simulink library "BilnrIntrpnMplXDyn"  (R2013b)
settings: Solver=ode45  StartTime=0.0  StopTime=10.0  RelTol=1e-3
settings Model: Creator=qzwc4r  LastModifiedBy=DZ1YRM

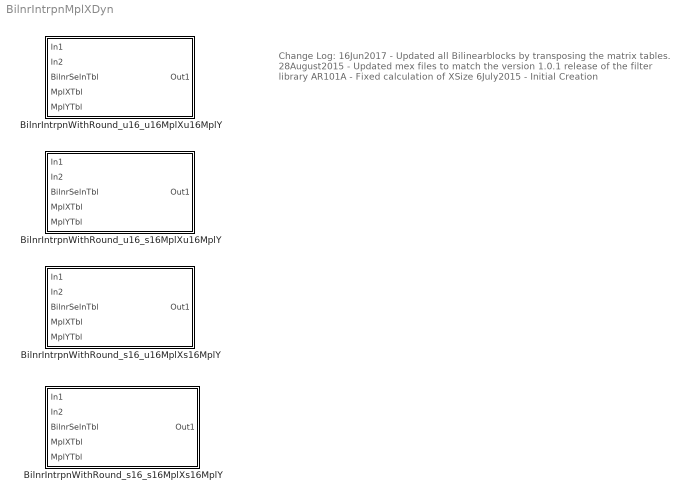
== system BilnrIntrpnMplXDyn ==
  note: Change Log:
      |
      | 16Jun2017
      | - Updated all Bilinearblocks by transposing the matrix tables.
      |
      | 28August2015
      | - Updated mex files to match the version 1.0.1 release of the filter library AR101A
      | - Fixed calculation of XSize
      |
      | 6July2015
      | - Initial Creation
  BilnrIntrpnWithRound_s16_s16MplXs16MplY : Subsystem  mask(BilnrIntrpnWithRound_s16_s16MplXs16MplY){}
      mask help: Bilinear interpolation with signed input and signed output (multiple X tables, multiple Y tables)
      settings: AttributesFormatString=Bilnr ( s16MplX , s16MplY )
      mask Display:
      | Xx = [0.45, .9];
      | Xy = [0.5, 0.5];
      | Yx = [0.6750, 0.6750];
      | Yy = [0.1, .9];
      | 
      | px = [.45, .5, .7, .75, .8, .9];
      | py1 = [.1,  .1, .3, .4, .5, .9];
      | py2 = py1+0.15;
      | py3 = py2+0.15;
      | plot(Xx,Xy, Yx,Yy, px,py1, px,py2, px,py3)
      | 
      | port_label('input',1,'Inp')
      | port_label('input',2,'BilnrSelInp')
      | port_label('input',3,'BilnrSelnTbl')
      | port_label('input',4,'MplXTbl')
      | port_label('input',5,'MplYTbl')
  BilnrIntrpnWithRound_s16_u16MplXs16MplY : Subsystem  mask(BilnrIntrpnWithRound_s16_u16MplXs16MplY){}
      mask help: Bilinear interpolation with unsigned input and signed output (multiple X tables, multiple Y tables)
      settings: AttributesFormatString=Bilnr ( u16MplX , s16MplY )
      mask Display:
      | Xx = [0.45, .9];
      | Xy = [0.4, 0.4];
      | Yx = [0.45, 0.45];
      | Yy = [0, .7];
      | 
      | px = [0.45, .5, .6, .7, .8, .9];
      | py1 = [.72, .7, .6, .3, .25, .25];
      | py2 = py1-0.1;
      | py3 = py2-0.1;
      | 
      | plot(Xx,Xy, Yx,Yy, px,py1, px,py2, px,py3)
      | 
      | port_label('input',1,'Inp')
      | port_label('input',2,'BilnrSelInp')
      | port_label('input',3,'BilnrSelnTbl')
      | port_label('input',4,'MplXTbl')
      | port_label('input',5,'MplYTbl')
  BilnrIntrpnWithRound_u16_s16MplXu16MplY : Subsystem  mask(BilnrIntrpnWithRound_u16_s16MplXu16MplY){}
      mask help: Bilinear interpolation with signed input and unsigned output (multiple X tables, multiple Y tables)
      settings: AttributesFormatString=Bilnr ( u16MplX , u16MplY )
      mask Display:
      | Xx = [.45, .9];
      | Xy = [.05, .05];
      | Yx = [.675, .675];
      | Yy = [.05, .9];
      | 
      | px = [0.45, .5, .6, .7, .8, .9];
      | py1 = [.1, .1, .2, .5, .6, .65];
      | py2 = py1+.15;
      | py3 = py2+.15;
      | 
      | plot(Xx,Xy, Yx,Yy, px,py1, px,py2, px,py3)
      | 
      | port_label('input',1,'Inp')
      | port_label('input',2,'BilnrSelInp')
      | port_label('input',3,'BilnrSelnTbl')
      | port_label('input',4,'MplXTbl')
      | port_label('input',5,'MplYTbl')
  BilnrIntrpnWithRound_u16_u16MplXu16MplY : Subsystem  mask(BilnrIntrpnWithRound_u16_u16MplXu16MplY){}
      mask help: Bilinear interpolation with signed input and unsigned output (multiple X tables, multiple Y tables)
      settings: AttributesFormatString=Bilnr ( u16MplX , u16MplY )
      mask Display:
      | Xx = [0.45, .9];
      | Xy = [0.1, 0.1];
      | Yx = [0.45, 0.45];
      | Yy = [0.1, .7];
      | 
      | px = [0.45, .5, .55, .6, .65, .7, .9];
      | 
      | py1 = [0.1,  0.4, .6, .7, .75, .8, .8];
      | py2 = [0.1,  0.4, .5, .6, .65, .7, .7];
      | py3 = [0.1,  0.3, .4, .5, .55, .6, .6];
      | 
      | plot(Xx,Xy, Yx,Yy, px,py1, px,py2, px,py3)
      | 
      | port_label('input',1,'Inp')
      | port_label('input',2,'BilnrSelInp')
      | port_label('input',3,'BilnrSelnTbl')
      | port_label('input',4,'MplXTbl')
      | port_label('input',5,'MplYTbl')

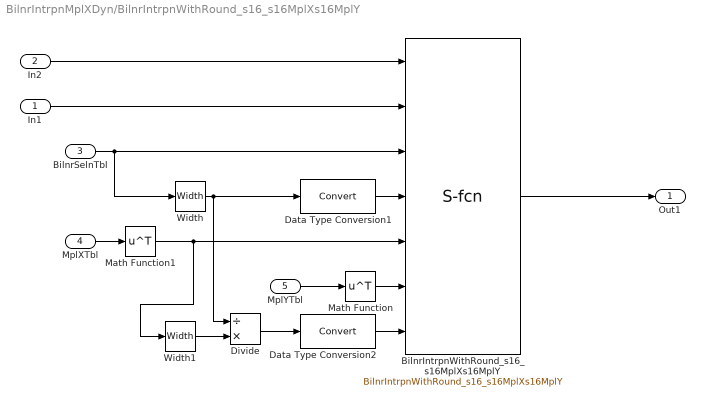
== system BilnrIntrpnMplXDyn/BilnrIntrpnWithRound_s16_s16MplXs16MplY ==
  In1 : Inport
  In2 : Inport  Port=2
  BilnrSelnTbl : Inport  Port=3
  MplXTbl : Inport  Port=4
  MplYTbl : Inport  Port=5
  BilnrIntrpnWithRound_s16_s16MplXs16MplY : S-Function  FunctionName=BilnrIntrpnWithRound_s16_s16MplXs16MplY  EnableBusSupport=off  mask(Legacy Function){SFunctionSpec=int16 y1 = BilnrIntrpnWithRound_s16_s16MplXs16MplY(uint16 u1,  int16 u2, uint16 u3[], uint16 u4,  int16 u5[],  int16 u6[], uint16 u7), ShowSpec=off}
      mask prompts: ShowSpec "Display function specification"
      mask help:
      | This block allows you to call the legacy functions specified by the following Legacy Code Tool definition:
      | def.SFunctionName = 'BilnrIntrpnWithRound_s16_s16MplXs16MplY';
      | def.OutputFcnSpec = ' int16 y1 = BilnrIntrpnWithRound_s16_s16MplXs16MplY(uint16 u1,  int16 u2, uint16 u3[], uint16 u4,  int16 u5[],  int16 u6[], uint16 u7)';
      | def.HeaderFiles = {'NxtrIntrpn.h', 'NxtrIntrpn_MemMap.h', 'Std_Types.h', 'Platform_Types.h', 'Compiler.h', 'Compiler_Cfg.h'};
      | def.SourceFiles = {'NxtrIntrpn.c'};
      | def.IncPaths = {'..\SrcFiles'};
      | def.SrcPaths = {'..\SrcFiles'};
      mask Help: <p>This block was generated automatically by the Legacy Code Tool. For detailed help on this tool, call<a href="matlab:legacy_code('help')"> legacy_code('help')</a>.</p>
      mask Callback ShowSpec:
      | if strcmp(get_param(gcbh, 'ShowSpec'), 'on')
      |   set_param(gcbh, 'MaskDisplay', sprintf('fprintf(''%s'');', get_param(gcbh, 'SFunctionSpec')));
      | else
      |   set_param(gcbh, 'MaskDisplay', sprintf('fprintf(''%s'');', get_param(gcbh, 'FunctionName')));
      | end
      mask Display: fprintf('%s',' int16 y1 = BilnrIntrpnWithRound_s16_s16MplXs16MplY(uint16 u1,  int16 u2, uint16 u3[], uint16 u4,  int16 u5[],  int16 u6[], uint16 u7)');
  Data Type Conversion1 : DataTypeConversion
  Data Type Conversion2 : DataTypeConversion
  Divide : Product  Inputs=/*
  Math Function : Math  Operator=transpose  SaturateOnIntegerOverflow=on
  Math Function1 : Math  Operator=transpose  SaturateOnIntegerOverflow=on
  Width : Width
  Width1 : Width
  Out1 : Outport
  wires:
  Width/1 -> Data Type Conversion1/1, Divide/1
  BilnrSelnTbl/1 -> Width/1, BilnrIntrpnWithRound_s16_s16MplXs16MplY/3
  In2/1 -> BilnrIntrpnWithRound_s16_s16MplXs16MplY/1
  MplYTbl/1 -> Math Function/1
  BilnrIntrpnWithRound_s16_s16MplXs16MplY/1 -> Out1/1
  In1/1 -> BilnrIntrpnWithRound_s16_s16MplXs16MplY/2
  Data Type Conversion1/1 -> BilnrIntrpnWithRound_s16_s16MplXs16MplY/4
  Data Type Conversion2/1 -> BilnrIntrpnWithRound_s16_s16MplXs16MplY/7
  MplXTbl/1 -> Math Function1/1
  Width1/1 -> Divide/2
  Divide/1 -> Data Type Conversion2/1
  Math Function/1 -> BilnrIntrpnWithRound_s16_s16MplXs16MplY/6
  Math Function1/1 -> BilnrIntrpnWithRound_s16_s16MplXs16MplY/5, Width1/1

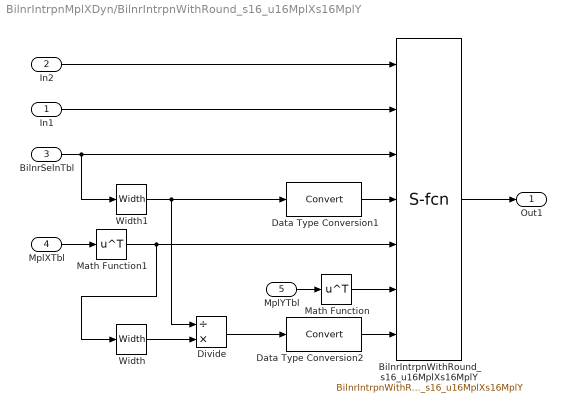
== system BilnrIntrpnMplXDyn/BilnrIntrpnWithRound_s16_u16MplXs16MplY ==
  In1 : Inport
  In2 : Inport  Port=2
  BilnrSelnTbl : Inport  Port=3
  MplXTbl : Inport  Port=4
  MplYTbl : Inport  Port=5
  BilnrIntrpnWithRound_s16_u16MplXs16MplY : S-Function  FunctionName=BilnrIntrpnWithRound_s16_u16MplXs16MplY  EnableBusSupport=off  mask(Legacy Function){SFunctionSpec=int16 y1 = BilnrIntrpnWithRound_s16_u16MplXs16MplY(uint16 u1, uint16 u2, uint16 u3[], uint16 u4, uint16 u5[],  int16 u6[], uint16 u7), ShowSpec=off}
      mask prompts: ShowSpec "Display function specification"
      mask help:
      | This block allows you to call the legacy functions specified by the following Legacy Code Tool definition:
      | def.SFunctionName = 'BilnrIntrpnWithRound_s16_u16MplXs16MplY';
      | def.OutputFcnSpec = ' int16 y1 = BilnrIntrpnWithRound_s16_u16MplXs16MplY(uint16 u1, uint16 u2, uint16 u3[], uint16 u4, uint16 u5[],  int16 u6[], uint16 u7)';
      | def.HeaderFiles = {'NxtrIntrpn.h', 'NxtrIntrpn_MemMap.h', 'Std_Types.h', 'Platform_Types.h', 'Compiler.h', 'Compiler_Cfg.h'};
      | def.SourceFiles = {'NxtrIntrpn.c'};
      | def.IncPaths = {'..\SrcFiles'};
      | def.SrcPaths = {'..\SrcFiles'};
      mask Help: <p>This block was generated automatically by the Legacy Code Tool. For detailed help on this tool, call<a href="matlab:legacy_code('help')"> legacy_code('help')</a>.</p>
      mask Callback ShowSpec:
      | if strcmp(get_param(gcbh, 'ShowSpec'), 'on')
      |   set_param(gcbh, 'MaskDisplay', sprintf('fprintf(''%s'');', get_param(gcbh, 'SFunctionSpec')));
      | else
      |   set_param(gcbh, 'MaskDisplay', sprintf('fprintf(''%s'');', get_param(gcbh, 'FunctionName')));
      | end
      mask Display: fprintf('%s',' int16 y1 = BilnrIntrpnWithRound_s16_u16MplXs16MplY(uint16 u1, uint16 u2, uint16 u3[], uint16 u4, uint16 u5[],  int16 u6[], uint16 u7)');
  Data Type Conversion1 : DataTypeConversion
  Data Type Conversion2 : DataTypeConversion
  Divide : Product  Inputs=/*
  Math Function : Math  Operator=transpose  SaturateOnIntegerOverflow=on
  Math Function1 : Math  Operator=transpose  SaturateOnIntegerOverflow=on
  Width : Width
  Width1 : Width
  Out1 : Outport
  wires:
  BilnrSelnTbl/1 -> BilnrIntrpnWithRound_s16_u16MplXs16MplY/3, Width1/1
  In2/1 -> BilnrIntrpnWithRound_s16_u16MplXs16MplY/1
  BilnrIntrpnWithRound_s16_u16MplXs16MplY/1 -> Out1/1
  In1/1 -> BilnrIntrpnWithRound_s16_u16MplXs16MplY/2
  Width1/1 -> Divide/1, Data Type Conversion1/1
  Data Type Conversion1/1 -> BilnrIntrpnWithRound_s16_u16MplXs16MplY/4
  Data Type Conversion2/1 -> BilnrIntrpnWithRound_s16_u16MplXs16MplY/7
  MplXTbl/1 -> Math Function1/1
  MplYTbl/1 -> Math Function/1
  Divide/1 -> Data Type Conversion2/1
  Width/1 -> Divide/2
  Math Function/1 -> BilnrIntrpnWithRound_s16_u16MplXs16MplY/6
  Math Function1/1 -> BilnrIntrpnWithRound_s16_u16MplXs16MplY/5, Width/1

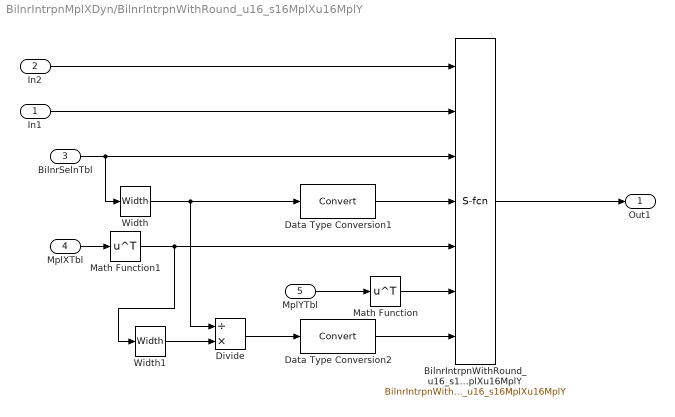
== system BilnrIntrpnMplXDyn/BilnrIntrpnWithRound_u16_s16MplXu16MplY ==
  In1 : Inport
  In2 : Inport  Port=2
  BilnrSelnTbl : Inport  Port=3
  MplXTbl : Inport  Port=4
  MplYTbl : Inport  Port=5
  BilnrIntrpnWithRound_u16_s16MplXu16MplY : S-Function  FunctionName=BilnrIntrpnWithRound_u16_s16MplXu16MplY  EnableBusSupport=off  mask(Legacy Function){SFunctionSpec=uint16 y1 = BilnrIntrpnWithRound_u16_s16MplXu16MplY(uint16 u1,  int16 u2, uint16 u3[], uint16 u4,  int16 u5[], uint16 u6[], uint16 u7), ShowSpec=off}
      mask prompts: ShowSpec "Display function specification"
      mask help:
      | This block allows you to call the legacy functions specified by the following Legacy Code Tool definition:
      | def.SFunctionName = 'BilnrIntrpnWithRound_u16_s16MplXu16MplY';
      | def.OutputFcnSpec = 'uint16 y1 = BilnrIntrpnWithRound_u16_s16MplXu16MplY(uint16 u1,  int16 u2, uint16 u3[], uint16 u4,  int16 u5[], uint16 u6[], uint16 u7)';
      | def.HeaderFiles = {'NxtrIntrpn.h', 'NxtrIntrpn_MemMap.h', 'Std_Types.h', 'Platform_Types.h', 'Compiler.h', 'Compiler_Cfg.h'};
      | def.SourceFiles = {'NxtrIntrpn.c'};
      | def.IncPaths = {'..\SrcFiles'};
      | def.SrcPaths = {'..\SrcFiles'};
      mask Help: <p>This block was generated automatically by the Legacy Code Tool. For detailed help on this tool, call<a href="matlab:legacy_code('help')"> legacy_code('help')</a>.</p>
      mask Callback ShowSpec:
      | if strcmp(get_param(gcbh, 'ShowSpec'), 'on')
      |   set_param(gcbh, 'MaskDisplay', sprintf('fprintf(''%s'');', get_param(gcbh, 'SFunctionSpec')));
      | else
      |   set_param(gcbh, 'MaskDisplay', sprintf('fprintf(''%s'');', get_param(gcbh, 'FunctionName')));
      | end
      mask Display: fprintf('%s','uint16 y1 = BilnrIntrpnWithRound_u16_s16MplXu16MplY(uint16 u1,  int16 u2, uint16 u3[], uint16 u4,  int16 u5[], uint16 u6[], uint16 u7)');
  Data Type Conversion1 : DataTypeConversion
  Data Type Conversion2 : DataTypeConversion
  Divide : Product  Inputs=/*
  Math Function : Math  Operator=transpose  SaturateOnIntegerOverflow=on
  Math Function1 : Math  Operator=transpose  SaturateOnIntegerOverflow=on
  Width : Width
  Width1 : Width
  Out1 : Outport
  wires:
  In1/1 -> BilnrIntrpnWithRound_u16_s16MplXu16MplY/2
  BilnrIntrpnWithRound_u16_s16MplXu16MplY/1 -> Out1/1
  In2/1 -> BilnrIntrpnWithRound_u16_s16MplXu16MplY/1
  BilnrSelnTbl/1 -> BilnrIntrpnWithRound_u16_s16MplXu16MplY/3, Width/1
  Width/1 -> Divide/1, Data Type Conversion1/1
  Data Type Conversion1/1 -> BilnrIntrpnWithRound_u16_s16MplXu16MplY/4
  Data Type Conversion2/1 -> BilnrIntrpnWithRound_u16_s16MplXu16MplY/7
  MplYTbl/1 -> Math Function/1
  MplXTbl/1 -> Math Function1/1
  Width1/1 -> Divide/2
  Divide/1 -> Data Type Conversion2/1
  Math Function/1 -> BilnrIntrpnWithRound_u16_s16MplXu16MplY/6
  Math Function1/1 -> BilnrIntrpnWithRound_u16_s16MplXu16MplY/5, Width1/1

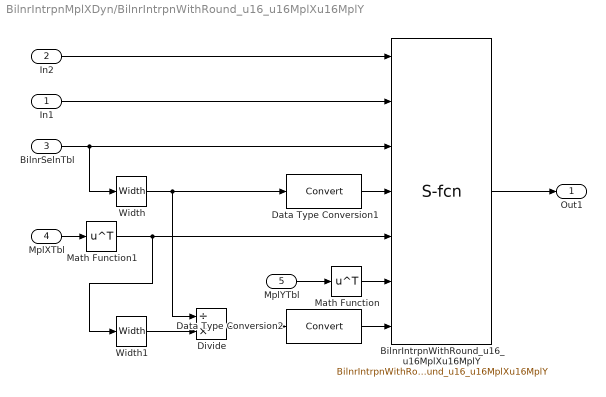
== system BilnrIntrpnMplXDyn/BilnrIntrpnWithRound_u16_u16MplXu16MplY ==
  In1 : Inport
  In2 : Inport  Port=2
  BilnrSelnTbl : Inport  Port=3
  MplXTbl : Inport  Port=4
  MplYTbl : Inport  Port=5
  BilnrIntrpnWithRound_u16_u16MplXu16MplY : S-Function  FunctionName=BilnrIntrpnWithRound_u16_u16MplXu16MplY  EnableBusSupport=off  mask(Legacy Function){SFunctionSpec=uint16 y1 = BilnrIntrpnWithRound_u16_u16MplXu16MplY(uint16 u1, uint16 u2, uint16 u3[], uint16 u4, uint16 u5[], uint16 u6[], uint16 u7), ShowSpec=off}
      mask prompts: ShowSpec "Display function specification"
      mask help:
      | This block allows you to call the legacy functions specified by the following Legacy Code Tool definition:
      | def.SFunctionName = 'BilnrIntrpnWithRound_u16_u16MplXu16MplY';
      | def.OutputFcnSpec = 'uint16 y1 = BilnrIntrpnWithRound_u16_u16MplXu16MplY(uint16 u1, uint16 u2, uint16 u3[], uint16 u4, uint16 u5[], uint16 u6[], uint16 u7)';
      | def.HeaderFiles = {'NxtrIntrpn.h', 'NxtrIntrpn_MemMap.h', 'Std_Types.h', 'Platform_Types.h', 'Compiler.h', 'Compiler_Cfg.h'};
      | def.SourceFiles = {'NxtrIntrpn.c'};
      | def.IncPaths = {'..\SrcFiles'};
      | def.SrcPaths = {'..\SrcFiles'};
      mask Help: <p>This block was generated automatically by the Legacy Code Tool. For detailed help on this tool, call<a href="matlab:legacy_code('help')"> legacy_code('help')</a>.</p>
      mask Callback ShowSpec:
      | if strcmp(get_param(gcbh, 'ShowSpec'), 'on')
      |   set_param(gcbh, 'MaskDisplay', sprintf('fprintf(''%s'');', get_param(gcbh, 'SFunctionSpec')));
      | else
      |   set_param(gcbh, 'MaskDisplay', sprintf('fprintf(''%s'');', get_param(gcbh, 'FunctionName')));
      | end
      mask Display: fprintf('%s','uint16 y1 = BilnrIntrpnWithRound_u16_u16MplXu16MplY(uint16 u1, uint16 u2, uint16 u3[], uint16 u4, uint16 u5[], uint16 u6[], uint16 u7)');
  Data Type Conversion1 : DataTypeConversion
  Data Type Conversion2 : DataTypeConversion
  Divide : Product  Inputs=/*
  Math Function : Math  Operator=transpose  SaturateOnIntegerOverflow=on
  Math Function1 : Math  Operator=transpose  SaturateOnIntegerOverflow=on
  Width : Width
  Width1 : Width
  Out1 : Outport
  wires:
  In1/1 -> BilnrIntrpnWithRound_u16_u16MplXu16MplY/2
  BilnrIntrpnWithRound_u16_u16MplXu16MplY/1 -> Out1/1
  In2/1 -> BilnrIntrpnWithRound_u16_u16MplXu16MplY/1
  BilnrSelnTbl/1 -> BilnrIntrpnWithRound_u16_u16MplXu16MplY/3, Width/1
  Width/1 -> Divide/1, Data Type Conversion1/1
  Data Type Conversion1/1 -> BilnrIntrpnWithRound_u16_u16MplXu16MplY/4
  Data Type Conversion2/1 -> BilnrIntrpnWithRound_u16_u16MplXu16MplY/7
  MplXTbl/1 -> Math Function1/1
  MplYTbl/1 -> Math Function/1
  Width1/1 -> Divide/2
  Divide/1 -> Data Type Conversion2/1
  Math Function/1 -> BilnrIntrpnWithRound_u16_u16MplXu16MplY/6
  Math Function1/1 -> BilnrIntrpnWithRound_u16_u16MplXu16MplY/5, Width1/1
